simulink model "CPMmodulator"  (Simulink 7.5)
settings: Solver=ode45  StartTime=0.0  StopTime=10.0  RelTol=1e-3
settings Model: Creator=rwe  LastModifiedBy=rwe

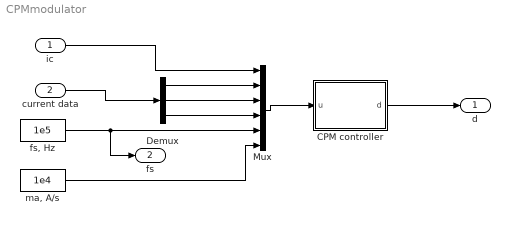
== system CPMmodulator ==
  ic : Inport  OutDataType=fixdt(1, 16)  OutScaling=2^0
  current data : Inport  Port=2  OutDataType=fixdt(1, 16)  OutScaling=2^0
  CPM controller : Stateflow chart  TreatAsAtomicUnit=on
  Demux : Demux  Outputs=3
  Mux : Mux  Inputs=6
  "fs, Hz" : Constant  Value=1e5  OutDataType=fixdt(1, 16)  OutScaling=2^0
  "ma, A/s" : Constant  Value=1e4  OutDataType=fixdt(1, 16)  OutScaling=2^0
  d : Outport  OutDataType=fixdt(1, 16)  OutScaling=2^0
  fs : Outport  Port=2  OutDataType=fixdt(1, 16)  OutScaling=2^0
  wires:
  Mux/1 -> CPM controller/1(u)
  ic/1 -> Mux/1
  CPM controller/1(d) -> d/1
  "fs, Hz"/1 -> fs/1, Mux/5
  "ma, A/s"/1 -> Mux/6
  current data/1 -> Demux/1
  Demux/1 -> Mux/2
  Demux/2 -> Mux/3
  Demux/3 -> Mux/4

== matlab function CPM controller ==
  data: u input double; d output double
function d = CPM(u)
%#eml
% Current mode controller, using Tan's model
% No sampling dynamics included
ic = u(1); % control current
i = u(2);  % average inductor current
m1 = u(3);  % inductor up slope
m2 = u(4);  % inductor down slope
fs = u(5);  % switching frequency
ma = u(6);  % slope of artificial ramp
b = ma/(m1+m2) + 0.5;
d = max(0,min(0.9,b*(1-sqrt(1-(ic-i)*2*fs/(m1+m2)/b^2)))); % duty cycle computation, including modulator saturation limits
